simulink model "mod_3R2010a"  (Simulink 7.5)
settings: Solver=ode45  StartTime=0.0  StopTime=10.0  RelTol=1e-3
settings Model: Creator=Professor Dingyu Xue  LastModifiedBy=Professor Dingyu Xue
settings OptimizationCC: InlineParams=on

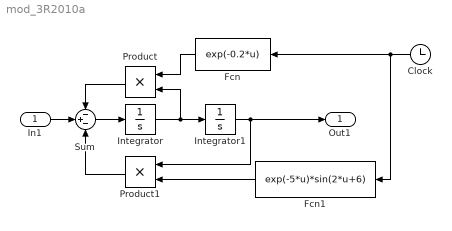
== system mod_3R2010a ==
  In1 : Inport
  Clock : Clock
  Fcn : Fcn  Expr=exp(-0.2*u)
  Fcn1 : Fcn  Expr=exp(-5*u)*sin(2*u+6)
  Integrator : Integrator
  Integrator1 : Integrator
  Product : Product  RndMeth=Zero
  Product1 : Product  RndMeth=Zero
  Sum : Sum  Inputs=-+-
  Out1 : Outport
  wires:
  Integrator/1 -> Integrator1/1, Product/2
  Sum/1 -> Integrator/1
  In1/1 -> Sum/2
  Integrator1/1 -> Out1/1, Product1/1
  Product/1 -> Sum/1
  Clock/1 -> Fcn/1, Fcn1/1
  Fcn/1 -> Product/1
  Fcn1/1 -> Product1/2
  Product1/1 -> Sum/3
